simulink model "automata_learning"  (R2022a)
settings: Solver=FixedStepAuto  StartTime=0.0  StopTime=10.0  FixedStep=0.005  RelTol=1e-3
settings Model: Creator=diego  LastModifiedBy=diego

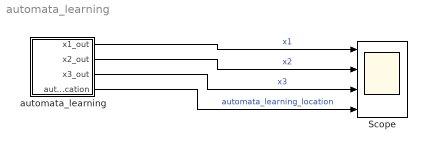
== system automata_learning ==
  Scope : Scope  NumInputPorts=4
  automata_learning : Stateflow chart  TreatAsAtomicUnit=on
  wires:
  automata_learning/1(x1_out) -> Scope/1  "x1"
  automata_learning/2(x2_out) -> Scope/2  "x2"
  automata_learning/3(x3_out) -> Scope/3  "x3"
  automata_learning/4(automata_learning_location) -> Scope/4  "automata_learning_location"

== stateflow chart automata_learning/automata_learning ==
  settings: updateMethod=CONTINUOUS
  state loc1
    du:
    x1_dot = 2.7431228543428006 - 4.6301046952285105 * x2 - 0.32975963571152533 * x3 - 5.762886537966551 * x1;
    x2_dot = 6.000051085837185 * x1 + 4.0000426370534115 * x2 + 0.9999675339204259 * x3 - 4.999981506232871;
    x3_dot = 3.0000258368527284 * x1 + 2.0000216435655602 * x2 - 2.500016514597519 * x3 + 0.5000095497398434;
    x1_out=x1;
    x2_out=x2;
    x3_out=x3;
    automata_learning_location =1;
  state loc2
    du:
    x1_dot = 2.200000402459409 * x1 + 3.6000004923407687 * x2 + 3.900000590569107 * x3 + 0.00000003061709207712905;
    x2_dot = 2.9619427530196845 * x1 + 2.3781141232102527 * x2 + 3.372186698274163 * x3 + 0.0011455256131647218;
    x3_dot = -5.0000005880283425 * x1 - 5.400000715846545 * x2 - 6.700000861121225 * x3 - 0.000000045978500107062004;
    x1_out=x1;
    x2_out=x2;
    x3_out=x3;
    automata_learning_location =2;
  loc1 -> loc2 : [3.613 * x1 + 3.088 * x2 - 2.026 * x3 + 1.0 > 0.0]
  (default) -> loc1 : {x1 = 0.0;
      | x2 = 0.0;
      | x3 = 0.0;}
  data: x1_out output; x1 local; x2_out output; x2 local; x3_out output; x3 local; automata_learning_location output
  data x1 settings: updateMethod=SF_CONTINUOUS_TIME_DATA
  data x2 settings: updateMethod=SF_CONTINUOUS_TIME_DATA
  data x3 settings: updateMethod=SF_CONTINUOUS_TIME_DATA
